simulink model "bldc_sim"  (R2012b)
settings: Solver=ode3  StartTime=0.0  StopTime=2.5  RelTol=1e-3
undefined symbols (not defined in the file or in its folder): DiscIntNeverNeededParam
libraries: simulink x7, powerlib x6, xbsIndex_r4 x1
settings Model: Creator=andrei  LastModifiedBy=andrei
settings DebuggingCC: SingleTaskRateTransMsg=error

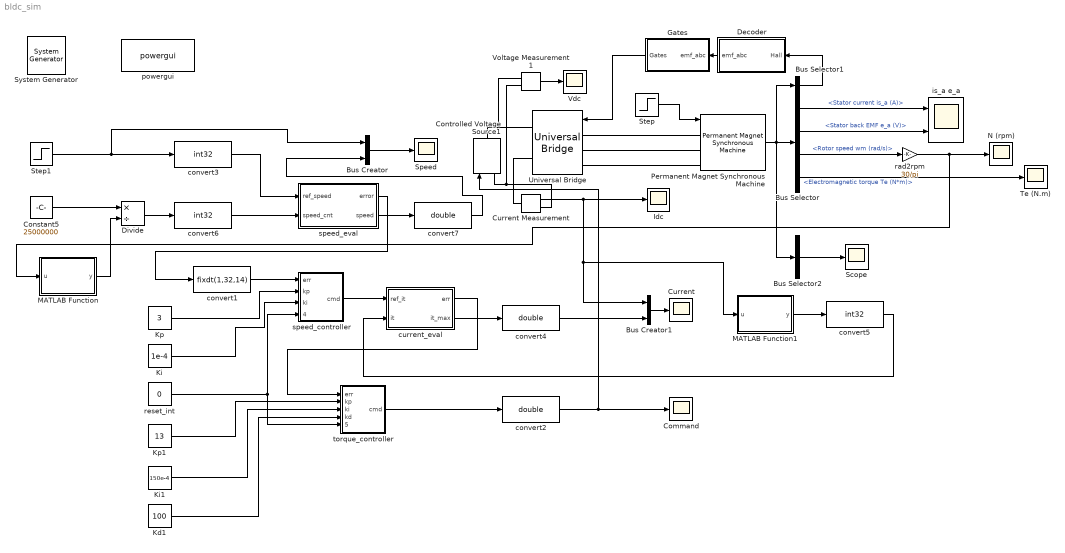
== system bldc_sim ==
  " System Generator" : xbsIndex_r4/ System Generator  Tag=genX  xilinxfamily=zynq  part=xc7z020  speed=-1  package=clg484  synthesis_tool=XST  clock_wrapper=Clock Enables  directory=./netlist  proj_type=Project Navigator  Synth_file=XST Defaults  Impl_file=ISE Defaults  testbench=off  simulink_period=1  sysclk_period=10  dcm_input_clock_period=10  incr_netlist=off  trim_vbits=Everywhere in SubSystem  dbl_ovrd=According to Block Masks  core_generation=According to Block Masks  run_coregen=off  deprecated_control=off  eval_field=0  block_type=sysgen
  Bus Selector : BusSelector  OutputSignals=Stator current is_a (A),Stator back EMF e_a (V),Rotor speed wm (rad/s),Electromagnetic torque Te (N*m)
  Bus Selector1 : BusSelector  OutputSignals=Hall effect signal h_a,Hall effect signal h_b,Hall effect signal h_c  OutputAsBus=on
  Bus Selector2 : BusSelector  OutputSignals=Stator current is_a (A),Stator current is_b (A),Stator current is_c (A)  OutputAsBus=on
  Bus Creator : BusCreator  Inputs=2
  Bus Creator1 : BusCreator  Inputs=2
  Command : Scope
      settings: TimeRange=0.2  YMin=30  YMax=150  SaveName=ScopeData5  DataFormat=Structure
  Constant5 : Constant  Value=25000000  OutDataTypeStr=double
  Controlled Voltage Source1 : powerlib/Electrical Sources/Controlled Voltage Source  Initialize=on  Source_Type=DC  Amplitude=0  Phase=0  Frequency=0  Measurements=None
  Current : Scope
      settings: TimeRange=0.2  YMin=-17.5  YMax=20  SaveName=ScopeData4  DataFormat=Structure
  Current Measurement : powerlib/Measurements/Current Measurement  PhasorSimulation=off  OutputType=Complex  PSBequivalent=0
  Decoder : Subsystem
  Divide : Product  Inputs=*/
  Gates : Subsystem
  Idc : Scope
      settings: TimeRange=0.2  YMin=-50  YMax=400  DataFormat=Structure
  Kd1 : Constant  Value=100  OutDataTypeStr=fixdt(1,32,14)
  Ki : Constant  Value=1e-4  OutDataTypeStr=fixdt(1,32,14)
  Ki1 : Constant  Value=150e-4  OutDataTypeStr=fixdt(1,32,14)
  Kp : Constant  Value=3  OutDataTypeStr=fixdt(1,32,14)
  Kp1 : Constant  Value=13  OutDataTypeStr=fixdt(1,32,14)
  MATLAB Function : MATLAB Function  TreatAsAtomicUnit=on
  MATLAB Function1 : MATLAB Function  TreatAsAtomicUnit=on
  N (rpm) : Scope
      settings: TimeRange=0.2  YMin=256  YMax=269  SaveName=N
  Permanent Magnet Synchronous Machine : powerlib/Machines/Permanent Magnet Synchronous Machine  NbPhases=3  FluxDistribution=Trapezoidal  RotorType=Round  MechanicalLoad=Torque Tm  PresetModel=No  ShowDetailedParameters=on  Resistance=1.8  Inductance=2.1e-3  dqInductances=[8.5e-3, 8.5e-3]  La=0.000835  MachineConstant=Torque Constant (N.m / A_peak)  Flux=0.0044135  VoltageCst=3.6974  TorqueCst=0.03530775916665  Flat=120  Mechanical=[ 0.8e-3 1e-3 4]  PolePairs=4  InitialConditions=[0,0, 0,0]  InitialConditions5ph=[0 0 0 0 0 0]  TsPowergui=0  TsBlock=-1  RefAngle=Aligned with phase A axis (original Park)
  Scope : Scope
      settings: SaveName=ScopeData2
  Speed : Scope
      settings: TimeRange=0.2  YMin=5000  YMax=5040  SaveName=ScopeData3  DataFormat=Structure
  Step : Step  Time=.4  After=0.2  SampleTime=0.00001
  Step1 : Step  Before=3000  After=5000  SampleTime=0.00001  ZeroCross=off
  Te (N.m) : Scope
      settings: TimeRange=0.2  YMin=0  YMax=3500  SaveName=N1
  Universal Bridge : powerlib/Power Electronics/Universal Bridge  Arms=3  SnubberResistance=5000  SnubberCapacitance=1e-6  Device=MOSFET / Diodes  Ron=1e-3  Lon=0  ForwardVoltages="[  0  0  ]"  ForwardVoltage=0  GTOparameters=[ 10e-6 , 20e-6 ]  IGBTparameters=[ 1e-6 , 2e-6 ]  Measurements=None  Measurements_2=None  converterType=Rectifier
  Vdc : Scope
      settings: TimeRange=0.2  YMin=60  YMax=110  DataFormat=Structure
  Voltage Measurement1 : powerlib/Measurements/Voltage Measurement  PhasorSimulation=off  OutputType=Complex  PSBequivalent=0
  convert1 : DataTypeConversion  OutDataTypeStr=fixdt(1,32,14)
  convert2 : DataTypeConversion  OutDataTypeStr=double
  convert3 : DataTypeConversion  OutDataTypeStr=int32  ConvertRealWorld=Stored Integer (SI)  LockScale=on
  convert4 : DataTypeConversion  OutDataTypeStr=double
  convert5 : DataTypeConversion  OutDataTypeStr=int32  ConvertRealWorld=Stored Integer (SI)  LockScale=on
  convert6 : DataTypeConversion  OutDataTypeStr=int32  ConvertRealWorld=Stored Integer (SI)  LockScale=on
  convert7 : DataTypeConversion  OutDataTypeStr=double
  current_eval : Subsystem
  is_a e_a : Scope  NumInputPorts=2
      settings: TimeRange=0.2  YMin=-15~-250  YMax=20~250  SaveName=IE
  powergui : powerlib/powergui  Priority=2  SimulationMode=Discrete  SolverType=Tustin  SampleTime=1e-5  frequency=60  SPID=off  DisableSnubberDevices=off  DisableRonSwitches=off  DisableVfSwitches=off  SwTol=0  Interpol=off  DisplayEquations=off  FunctionMessages=off  frequencyindice=0  Pbase=100e6  ErrMax=1e-4  Iterations=50  UnitsV=kV  UnitsW=MW  echomessages=off  HookPort=off  EnableUseOfTLC=off  x0status=blocks  RestoreLinks=warning  ResistiveCurrentMeasurement=off  Frange=[0:2:500]  Ylog=off  Xlog=on  ShowGrid=off  save=off  variable=ZData  ZoomFFT=on  StartTime=0.0  cycles=1  DisplayStyle=1  fundamental=60  FreqAxis=off  MaxFrequency=1000  frequencyindicesteady=1  RmsSteady=1  display=off  Ts=0  methode=off
  rad2rpm : Gain  Gain=30/pi
  reset_int : Constant  Value=0  OutDataTypeStr=boolean
  speed_controller : Subsystem
  speed_eval : Subsystem
  torque_controller : Subsystem
  wires:
  Step/1 -> Permanent Magnet Synchronous Machine/1
  Gates/1(Gates) -> Universal Bridge/1
  Decoder/1(emf_abc) -> Gates/1("emf_abc ")
  rad2rpm/1 -> MATLAB Function/1(u), N (rpm)/1
  Voltage Measurement1/1 -> Vdc/1
  Bus Selector/1 -> is_a e_a/1  "<Stator current is_a (A)>"
  Permanent Magnet Synchronous Machine/1 -> Bus Selector2/1, Bus Selector/1, Bus Selector1/1
  Bus Selector1/1 -> Decoder/1("Hall ")
  Bus Selector/2 -> is_a e_a/2  "<Stator back EMF e_a (V)>"
  Bus Selector/3 -> rad2rpm/1  "<Rotor speed wm (rad/s)>"
  Bus Selector/4 -> Te (N.m)/1  "<Electromagnetic torque Te (N*m)>"
  Bus Selector2/1 -> Scope/1
  Constant5/1 -> Divide/1
  speed_eval/1(error) -> convert1/1
  Bus Creator/1 -> Speed/1
  convert1/1 -> speed_controller/1(err)
  Kp/1 -> speed_controller/2(kp)
  Ki/1 -> speed_controller/3(ki)
  reset_int/1 -> torque_controller/5(reset_int), speed_controller/4(reset_int)
  Bus Creator1/1 -> Current/1
  Kd1/1 -> torque_controller/4(kd)
  torque_controller/1(cmd) -> convert2/1
  Kp1/1 -> torque_controller/2(kp)
  Ki1/1 -> torque_controller/3(ki)
  current_eval/1(err) -> torque_controller/1(err)
  speed_controller/1(cmd) -> current_eval/1(ref_it)
  convert4/1 -> Bus Creator1/2
  Current Measurement/1 -> Bus Creator1/1, MATLAB Function1/1(u), Idc/1
  Step1/1 -> Bus Creator/1, convert3/1
  Divide/1 -> convert6/1
  speed_eval/2(speed) -> convert7/1
  convert7/1 -> Bus Creator/2
  MATLAB Function/1(y) -> Divide/2
  convert3/1 -> speed_eval/1(ref_speed)
  convert6/1 -> speed_eval/2(speed_cnt)
  convert5/1 -> current_eval/2(it)
  MATLAB Function1/1(y) -> convert5/1
  current_eval/2(it_max) -> convert4/1
  convert2/1 -> Command/1, Controlled Voltage Source1/1
  connections:
  Universal Bridge/LConn1 -- Permanent Magnet Synchronous Machine/LConn1
  Universal Bridge/LConn2 -- Permanent Magnet Synchronous Machine/LConn2
  Voltage Measurement1/LConn1 -- Controlled Voltage Source1/RConn1 -- Universal Bridge/RConn1
  Controlled Voltage Source1/LConn1 -- Current Measurement/RConn1 -- Voltage Measurement1/LConn2
  Universal Bridge/LConn3 -- Permanent Magnet Synchronous Machine/LConn3
  Universal Bridge/RConn2 -- Current Measurement/LConn1

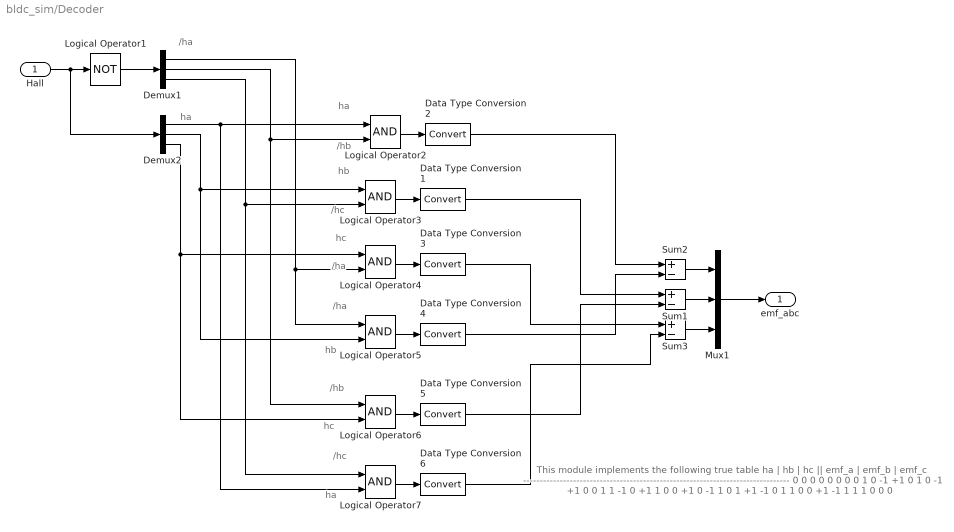
== system bldc_sim/Decoder ==
  note: /ha
  note: ha
  note: ha
  note: /hb
  note: hb
  note: /hc
  note: hc
  note: /ha
  note: /ha
  note: hb
  note: /hb
  note: hc
  note: /hc
  note: ha
  note: This module implements the following true table
      |
      |    ha   |   hb   |   hc   ||   emf_a   |   emf_b   |   emf_c
      |     --------------------------------------------------------------------------------
      | 0          0         0          0               0               0
      | 0          0         1          0               -1              +1
      | 0          1         0          -1              +1                0
      | 0          1         1          -1               0               +1
      | 1          0         0         +1               0               -1
      | 1          0         1         +1              -1                0
      | 1          1         0          0              +1               -1
      | 1          1         1          0               0                0
  "Hall " : Inport
  Data Type Conversion{1..6} (6 alike) : DataTypeConversion
  Demux1 : Demux  Outputs=3
  Demux2 : Demux  Outputs=3
  Logical Operator1 : Logic  Operator=NOT  AllPortsSameDT=off  OutDataTypeStr=boolean
  Logical Operator{2..7} (6 alike) : Logic  AllPortsSameDT=off  OutDataTypeStr=boolean
  Mux1 : Mux  Inputs=3
  Sum1 : Sum  Inputs=+-  OutDataTypeStr=double
  Sum2 : Sum  Inputs=+-  OutDataTypeStr=double
  Sum3 : Sum  Inputs=+-  OutDataTypeStr=double
  emf_abc : Outport
  wires:
  "Hall "/1 -> Logical Operator1/1, Demux2/1
  Logical Operator1/1 -> Demux1/1
  Demux2/3 -> Logical Operator4/1, Logical Operator6/2
  Demux2/2 -> Logical Operator3/1, Logical Operator5/2
  Demux2/1 -> Logical Operator2/1, Logical Operator7/2
  Demux1/3 -> Logical Operator3/2, Logical Operator7/1
  Demux1/2 -> Logical Operator2/2, Logical Operator6/1
  Demux1/1 -> Logical Operator4/2, Logical Operator5/1
  Logical Operator2/1 -> Data Type Conversion2/1
  Sum2/1 -> Mux1/1
  Sum1/1 -> Mux1/2
  Sum3/1 -> Mux1/3
  Mux1/1 -> emf_abc/1
  Logical Operator3/1 -> Data Type Conversion1/1
  Logical Operator4/1 -> Data Type Conversion3/1
  Logical Operator5/1 -> Data Type Conversion4/1
  Logical Operator6/1 -> Data Type Conversion5/1
  Logical Operator7/1 -> Data Type Conversion6/1
  Data Type Conversion2/1 -> Sum2/1
  Data Type Conversion4/1 -> Sum2/2
  Data Type Conversion1/1 -> Sum1/1
  Data Type Conversion5/1 -> Sum1/2
  Data Type Conversion3/1 -> Sum3/1
  Data Type Conversion6/1 -> Sum3/2

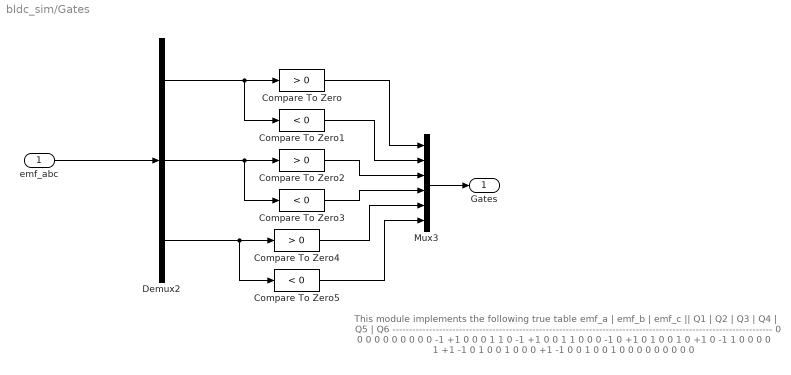
== system bldc_sim/Gates ==
  note: This module implements the following true table
      |
      |    emf_a   |   emf_b   |   emf_c   ||   Q1   |   Q2   |   Q3   |   Q4   |   Q5   |   Q6
      |     ------------------------------------------------------------------------------------------------------------------
      |       0              0                0            0          0          0           0        0        0
      |       0               -1              +1          0          0          0           1        1        0
      |     -1              +1                0          0          1          1           0        0        0
      |     -1               0               +1          0          1         0           0        1        0
      |    +1               0                -1          1          0          0           0        0        1
      |    +1              -1                0           1          0          0           1        0        0
      |      0              +1               -1           0          0          1           0        0        1
      |     0              0                0             0          0          0           0        0        0
  "emf_abc " : Inport
  Compare To Zero : simulink/Logic and Bit Operations/Compare To Zero  relop=>  OutDataTypeStr=boolean  ZeroCross=off
  Compare To Zero1 : simulink/Logic and Bit Operations/Compare To Zero  relop=<  OutDataTypeStr=boolean  ZeroCross=off
  Compare To Zero2 : simulink/Logic and Bit Operations/Compare To Zero  relop=>  OutDataTypeStr=boolean  ZeroCross=off
  Compare To Zero3 : simulink/Logic and Bit Operations/Compare To Zero  relop=<  OutDataTypeStr=boolean  ZeroCross=off
  Compare To Zero4 : simulink/Logic and Bit Operations/Compare To Zero  relop=>  OutDataTypeStr=boolean  ZeroCross=off
  Compare To Zero5 : simulink/Logic and Bit Operations/Compare To Zero  relop=<  OutDataTypeStr=boolean  ZeroCross=off
  Demux2 : Demux  Outputs=3
  Mux3 : Mux  Inputs=6
  Gates : Outport
  wires:
  "emf_abc "/1 -> Demux2/1
  Mux3/1 -> Gates/1
  Demux2/1 -> Compare To Zero/1, Compare To Zero1/1
  Demux2/2 -> Compare To Zero2/1, Compare To Zero3/1
  Demux2/3 -> Compare To Zero4/1, Compare To Zero5/1
  Compare To Zero/1 -> Mux3/1
  Compare To Zero1/1 -> Mux3/2
  Compare To Zero2/1 -> Mux3/3
  Compare To Zero3/1 -> Mux3/4
  Compare To Zero4/1 -> Mux3/5
  Compare To Zero5/1 -> Mux3/6

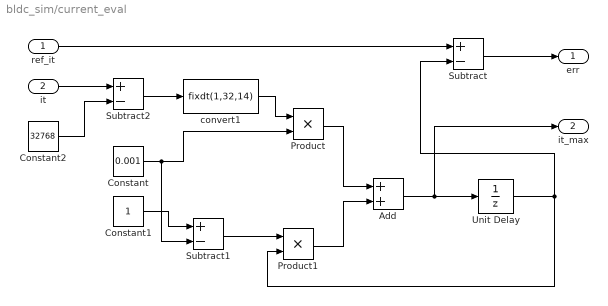
== system bldc_sim/current_eval ==
  ref_it : Inport  OutDataTypeStr=fixdt(1,32,14)  LockScale=on
  it : Inport  Port=2  OutDataTypeStr=fixdt(1,32,0)  LockScale=on
  Add : Sum  OutDataTypeStr=fixdt(1,32,14)  LockScale=on
  Constant : Constant  Value=0.001  OutDataTypeStr=fixdt(1,32,14)  SampleTime=-1  LockScale=on
  Constant1 : Constant  OutDataTypeStr=fixdt(1,32,14)  SampleTime=-1  LockScale=on
  Constant2 : Constant  Value=32768  OutDataTypeStr=fixdt(1,32,0)  SampleTime=-1  LockScale=on
  Product : Product  OutDataTypeStr=fixdt(1,32,14)  RndMeth=Zero  LockScale=on
  Product1 : Product  OutDataTypeStr=fixdt(1,32,14)  RndMeth=Zero  LockScale=on
  Subtract : Sum  Inputs=+-  OutDataTypeStr=fixdt(1,32,14)  LockScale=on
  Subtract1 : Sum  Inputs=+-  OutDataTypeStr=fixdt(1,32,14)  LockScale=on
  Subtract2 : Sum  Inputs=+-
  Unit Delay : UnitDelay  SampleTime=-1
  convert1 : DataTypeConversion  OutDataTypeStr=fixdt(1,32,14)  LockScale=on
  err : Outport  OutDataTypeStr=fixdt(1,32,14)  LockScale=on
  it_max : Outport  Port=2  OutDataTypeStr=fixdt(1,32,14)  LockScale=on
  wires:
  Subtract/1 -> err/1
  Constant/1 -> Subtract1/2, Product/2
  Constant1/1 -> Subtract1/1
  Subtract1/1 -> Product1/1
  Product/1 -> Add/1
  Product1/1 -> Add/2
  Add/1 -> Unit Delay/1, it_max/1
  ref_it/1 -> Subtract/1
  Unit Delay/1 -> Product1/2, Subtract/2
  convert1/1 -> Product/1
  it/1 -> Subtract2/1
  Subtract2/1 -> convert1/1
  Constant2/1 -> Subtract2/2

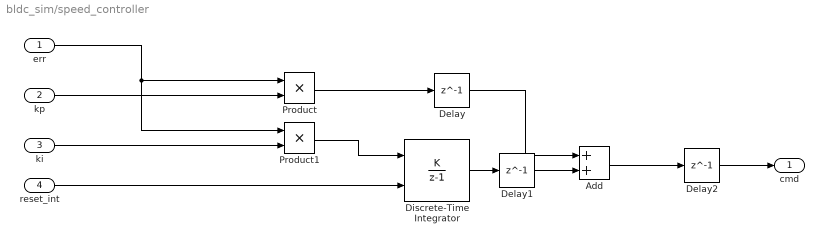
== system bldc_sim/speed_controller ==
  err : Inport  OutDataTypeStr=fixdt(1,32,14)  LockScale=on
  kp : Inport  Port=2  OutDataTypeStr=fixdt(1,32,14)  LockScale=on
  ki : Inport  Port=3  OutDataTypeStr=fixdt(1,32,14)  LockScale=on
  reset_int : Inport  Port=4  OutDataTypeStr=boolean  LockScale=on
  Add : Sum  AccumDataTypeStr=fixdt(1,32,14)  OutDataTypeStr=fixdt(1,32,14)  InputSameDT=on  LockScale=on
  Delay : Delay  DelayLength=1
  Delay1 : Delay  DelayLength=1
  Delay2 : Delay  DelayLength=1
  Discrete-Time Integrator : DiscreteIntegrator  IntegratorMethod=Accumulation: Forward Euler  gainval=1  ExternalReset=level  SampleTime=-1  OutDataTypeStr=fixdt(1,32,14)  LimitOutput=on  UpperSaturationLimit=12288  LowerSaturationLimit=0  ICPrevOutput=DiscIntNeverNeededParam  ICPrevScaledInput=DiscIntNeverNeededParam
      settings: LockScale=on
  Product : Product  OutDataTypeStr=fixdt(1,32,14)  SaturateOnIntegerOverflow=on  RndMeth=Zero  LockScale=on
  Product1 : Product  OutDataTypeStr=fixdt(1,32,14)  SaturateOnIntegerOverflow=on  RndMeth=Zero  LockScale=on
  cmd : Outport  OutDataTypeStr=fixdt(1,32,14)  LockScale=on
  wires:
  Product/1 -> Delay/1
  err/1 -> Product1/1, Product/1
  kp/1 -> Product/2
  ki/1 -> Product1/2
  Product1/1 -> Discrete-Time Integrator/1
  reset_int/1 -> Discrete-Time Integrator/2
  Add/1 -> Delay2/1
  Discrete-Time Integrator/1 -> Delay1/1
  Delay/1 -> Add/1
  Delay1/1 -> Add/2
  Delay2/1 -> cmd/1

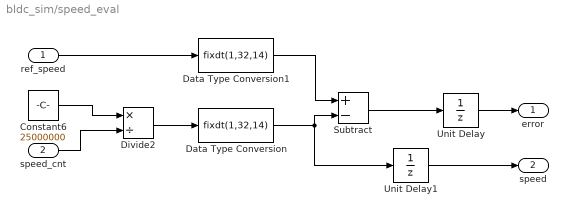
== system bldc_sim/speed_eval ==
  ref_speed : Inport  OutDataTypeStr=fixdt(1,32,0)  LockScale=on
  speed_cnt : Inport  Port=2  OutDataTypeStr=fixdt(1,32,0)  LockScale=on
  Constant6 : Constant  Value=25000000  OutDataTypeStr=fixdt(1,32,0)  LockScale=on
  Data Type Conversion : DataTypeConversion  OutDataTypeStr=fixdt(1,32,14)  LockScale=on
  Data Type Conversion1 : DataTypeConversion  OutDataTypeStr=fixdt(1,32,14)  LockScale=on
  Divide2 : Product  Inputs=*/  RndMeth=Simplest  SaturateOnIntegerOverflow=on  LockScale=on
  Subtract : Sum  Inputs=+-  OutDataTypeStr=fixdt(1,32,14)  LockScale=on
  Unit Delay : UnitDelay  SampleTime=-1
  Unit Delay1 : UnitDelay  SampleTime=-1
  error : Outport  OutDataTypeStr=fixdt(1,32,14)  LockScale=on
  speed : Outport  Port=2  OutDataTypeStr=fixdt(1,32,14)  LockScale=on
  wires:
  Constant6/1 -> Divide2/1
  ref_speed/1 -> Data Type Conversion1/1
  speed_cnt/1 -> Divide2/2
  Subtract/1 -> Unit Delay/1
  Divide2/1 -> Data Type Conversion/1
  Data Type Conversion/1 -> Subtract/2, Unit Delay1/1
  Unit Delay/1 -> error/1
  Unit Delay1/1 -> speed/1
  Data Type Conversion1/1 -> Subtract/1

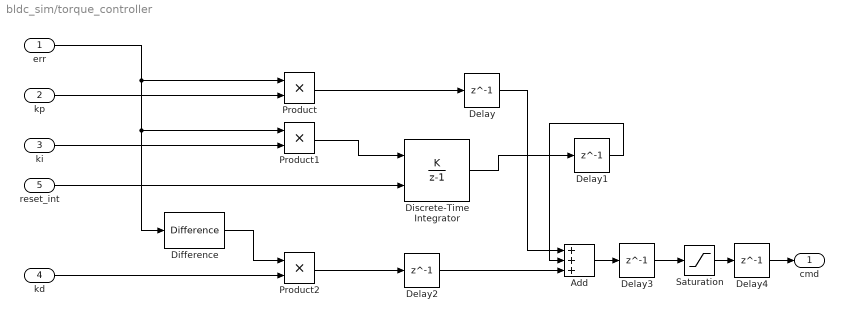
== system bldc_sim/torque_controller ==
  err : Inport  OutDataTypeStr=fixdt(1,32,14)  LockScale=on
  kp : Inport  Port=2  OutDataTypeStr=fixdt(1,32,14)  LockScale=on
  ki : Inport  Port=3  OutDataTypeStr=fixdt(1,32,14)  LockScale=on
  kd : Inport  Port=4  OutDataTypeStr=fixdt(1,32,14)  LockScale=on
  reset_int : Inport  Port=5  OutDataTypeStr=boolean  LockScale=on
  Add : Sum  Inputs=+++  AccumDataTypeStr=fixdt(1,32,14)  OutDataTypeStr=fixdt(1,32,14)  InputSameDT=on  LockScale=on
  Delay{,1..4} (5 alike) : Delay  DelayLength=1
  Difference : simulink/Discrete/Difference  ICPrevInput=0.0  InputProcessing=Inherited  OutMin=[]  OutMax=[]  OutDataTypeStr=fixdt(1,32,14)  OutputDataTypeScalingMode=Specify via dialog  OutDataType=fixdt(1,32,14)  OutScaling=[]  DoSatur=off
      settings: LockScale=on
  Discrete-Time Integrator : DiscreteIntegrator  IntegratorMethod=Accumulation: Forward Euler  gainval=1  ExternalReset=level  SampleTime=-1  OutDataTypeStr=fixdt(1,32,14)  LimitOutput=on  UpperSaturationLimit=2047  LowerSaturationLimit=0  ICPrevOutput=DiscIntNeverNeededParam  ICPrevScaledInput=DiscIntNeverNeededParam
      settings: LockScale=on
  Product : Product  OutDataTypeStr=fixdt(1,32,14)  RndMeth=Zero  LockScale=on
  Product1 : Product  OutDataTypeStr=fixdt(1,32,14)  RndMeth=Zero  LockScale=on
  Product2 : Product  OutDataTypeStr=fixdt(1,32,14)  RndMeth=Zero  LockScale=on
  Saturation : Saturate  UpperLimit=2047  LowerLimit=0  OutDataTypeStr=fixdt(1,32,14)
      settings: LockScale=on
  cmd : Outport  OutDataTypeStr=fixdt(1,32,14)  LockScale=on
  wires:
  Product/1 -> Delay/1
  err/1 -> Difference/1, Product1/1, Product/1
  kp/1 -> Product/2
  ki/1 -> Product1/2
  Product1/1 -> Discrete-Time Integrator/1
  reset_int/1 -> Discrete-Time Integrator/2
  Difference/1 -> Product2/1
  kd/1 -> Product2/2
  Product2/1 -> Delay2/1
  Add/1 -> Delay3/1
  Saturation/1 -> Delay4/1
  Delay/1 -> Add/1
  Discrete-Time Integrator/1 -> Delay1/1
  Delay1/1 -> Add/2
  Delay2/1 -> Add/3
  Delay3/1 -> Saturation/1
  Delay4/1 -> cmd/1

== matlab function bldc_sim/MATLAB Function1 ==
  data: u input; y output
function y = fcn(u)
%#codegen
y = u + 32768;

== matlab function bldc_sim/MATLAB Function ==
  data: u input; y output
function y = fcn(u)
%#codegen
y = u;
if(u == 0)
    y = 0.001;
end
